simulink model "sim_bank_and_economy"  (R2020a)
settings: Solver=VariableStepAuto  StartTime=0.0  StopTime=10.0  RelTol=1e-3
values from neighbouring files (symbols this model uses):
  c_fi = 0.5    [a_1.m]    (also in a_2.m; a_loss_function.m; bank_and_economy.m = 0.25)
  i_k = 0.06    [a_1.m]    (also in a_loss_function.m = 0.04; bank_and_economy.m = 0.04; full_model.m = 0.04)
  i_l = 0.075    [bank_and_economy.m]    (also in bank_centralbank.m = 0.055; bootstrapping.m = 0.055; main.m = 0.055)
  i_m = 0.03    [bank_and_economy.m]    (also in bank_centralbank.m; bootstrapping.m; main.m)
  K_0 = 0.08    [a_1.m]    (also in a_2.m; a_loss_function.m; bank_and_economy.m; bank_centralbank.m)
  K_p = 15    [a_1.m]    (also in a_2.m; a_loss_function.m; bank_and_economy.m = 0.5; bank_centralbank.m)
  l_k = 0.005    [bank_and_economy.m]
  lambda = 0.002    [a_1.m]    (also in a_2.m; a_loss_function.m; bank_and_economy.m; bank_centralbank.m)
  R = 1    [a_1.m]    (also in a_2.m; a_loss_function.m; bank_and_economy.m; bank_centralbank.m)
  r_k = 0.1    [a_1.m]    (also in a_2.m; a_loss_function.m; bank_and_economy.m; full_model.m)
  rate = 0.1    [a_1.m]    (also in a_2.m; a_loss_function.m; bank_and_economy.m; bank_centralbank.m)
  s_kf = 0.75    [bank_and_economy.m]
  sigma = 0.28    [a_1.m]    (also in a_2.m; a_loss_function.m; bank_and_economy.m; bank_centralbank.m)
  start_f = temp    (= 1)    [bank_and_economy.m]    (also in economy.m = 100)
  start_g = temp    (= 1)    [bank_and_economy.m]    (also in economy.m = 100)
  start_h = temp    (= 1)    [bank_and_economy.m]    (also in economy.m = 100)
  T_f = 0.5    [a_1.m]    (also in a_2.m; a_loss_function.m; bank_and_economy.m; bank_centralbank.m)
  T_g = 1    [a_1.m]    (also in a_2.m; a_loss_function.m; bank_and_economy.m; bank_centralbank.m)
  T_h = 0.1    [a_1.m]    (also in a_2.m; a_loss_function.m; bank_and_economy.m; bank_centralbank.m)
  T_i = 8    [a_1.m]    (also in a_2.m; a_loss_function.m; bank_and_economy.m; bank_centralbank.m)
  T_k = 0.1    [a_1.m]    (also in a_2.m; a_loss_function.m; bank_and_economy.m = 0.25; economy.m = 1)
  T_kf = 0.25    [bank_and_economy.m]
  tx = 0.3    [a_1.m]    (also in a_2.m; a_loss_function.m; bank_and_economy.m = 0.5; bank_centralbank.m = 0.25)
settings Model: Creator=erlended  LastModifiedBy=erlended

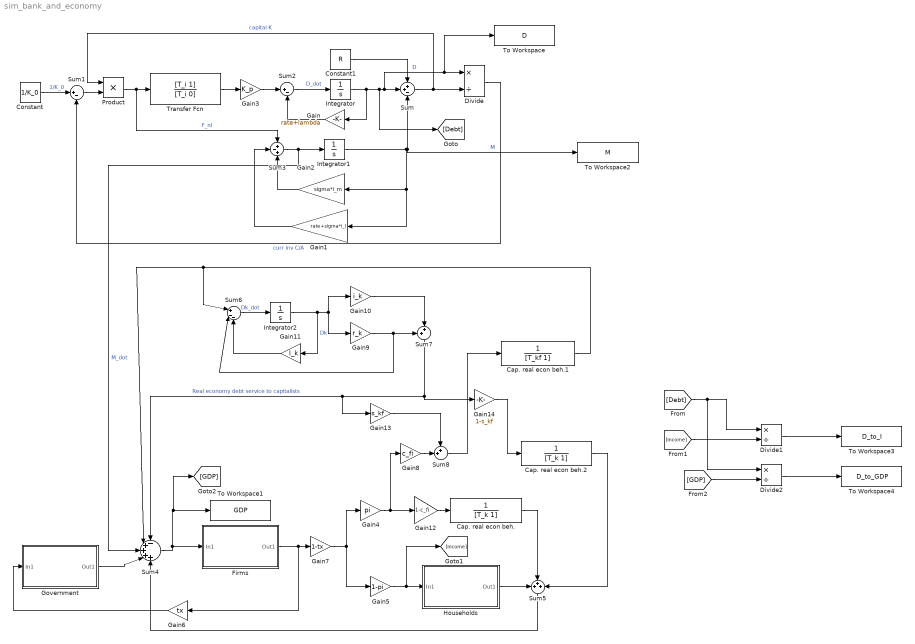
== system sim_bank_and_economy ==
  Cap. real econ beh. : TransferFcn  Denominator=[T_k 1]
  Cap. real econ beh.1 : TransferFcn  Denominator=[T_kf 1]
  Cap. real econ beh.2 : TransferFcn  Denominator=[T_k 1]
  Constant : Constant  Value=1/K_0
  Constant1 : Constant  Value=R
  Divide : Product  Inputs=*/
  Divide1 : Product  Inputs=*/
  Divide2 : Product  Inputs=*/
  Firms : Subsystem
  Gain : Gain  Gain=rate+lambda
  Gain1 : Gain  Gain=rate+sigma*i_l
  Gain10 : Gain  Gain=i_k
  Gain11 : Gain  Gain=l_k
  Gain12 : Gain  Gain=1-c_fi
  Gain13 : Gain  Gain=s_kf
  Gain14 : Gain  Gain=1-s_kf
  Gain2 : Gain  Gain=sigma*i_m
  Gain3 : Gain  Gain=K_p
  Gain4 : Gain  Gain=pi
  Gain5 : Gain  Gain=1-pi
  Gain6 : Gain  Gain=tx
  Gain7 : Gain  Gain=1-tx
  Gain8 : Gain  Gain=c_fi
  Gain9 : Gain  Gain=r_k
  Government : Subsystem
  Households : Subsystem
  Integrator : Integrator
  Integrator1 : Integrator
  Integrator2 : Integrator
  Product : Product
  Sum : Sum  Inputs=++-
  Sum1 : Sum  Inputs=|+-
  Sum2 : Sum  Inputs=|+-
  Sum3 : Sum  Inputs=+-+
  Sum4 : Sum  Inputs=-++++
  Sum5 : Sum  Inputs=+++
  Sum6 : Sum  Inputs=|+--
  Sum7 : Sum  Inputs=++|
  Sum8 : Sum  Inputs=++|
  To Workspace : ToWorkspace  VariableName=D  SaveFormat=Timeseries  SampleTime=-1
  To Workspace1 : ToWorkspace  VariableName=GDP  SaveFormat=Timeseries  SampleTime=-1
  To Workspace2 : ToWorkspace  VariableName=M  SaveFormat=Timeseries  SampleTime=-1
  To Workspace3 : ToWorkspace  VariableName=D_to_I  SaveFormat=Timeseries  SampleTime=-1
  To Workspace4 : ToWorkspace  VariableName=D_to_GDP  SaveFormat=Timeseries  SampleTime=-1
  Transfer Fcn : TransferFcn  Numerator=[T_i 1]  Denominator=[T_i 0]
  wires:
  Gain3/1 -> Sum2/1
  Integrator/1 -> Gain/1, [Debt], To Workspace/1, Divide/1, Sum/2  "D"
  Transfer Fcn/1 -> Gain3/1
  Divide/1 -> Sum1/2  "curr inv C/A"
  Gain1/1 -> Sum3/2
  Gain2/1 -> Sum3/3
  Sum1/1 -> Product/2
  Constant/1 -> Sum1/1  "1/K_0"
  Integrator1/1 -> Gain1/1, Gain2/1, To Workspace2/1, Sum/3  "M"
  Sum3/1 -> Sum4/3, Integrator1/1  "M_dot"
  Sum2/1 -> Integrator/1  "D_dot"
  Gain/1 -> Sum2/2
  Constant1/1 -> Sum/1
  Sum/1 -> Product/1, Divide/2  "capital K"
  Product/1 -> Transfer Fcn/1, Sum3/1  "F_nl"
  Households/1(Out1) -> Sum5/1
  Gain7/1 -> Gain4/1, Gain5/1
  Sum4/1 -> Firms/1(In1), [GDP], To Workspace1/1
  Sum5/1 -> Sum4/5
  Gain6/1 -> Government/1(In1)
  Firms/1(Out1) -> Gain7/1, Gain6/1
  Government/1(Out1) -> Sum4/4
  Gain5/1 -> [Income], Households/1(In1)
  Cap. real econ beh./1 -> Sum5/2
  Divide1/1 -> To Workspace3/1
  Divide2/1 -> To Workspace4/1
  [Debt] -> Divide1/1, Divide2/1
  [GDP] -> Divide2/2
  [Income] -> Divide1/2
  Integrator2/1 -> Gain11/1, Gain9/1, Gain10/1  "Dk"
  Sum6/1 -> Integrator2/1  "Dk_dot"
  Gain11/1 -> Sum6/3
  Gain10/1 -> Sum7/2
  Gain9/1 -> Sum6/2, Sum7/1
  Sum7/1 -> Gain14/1, Sum4/1, Gain13/1  "Real economy debt service to capitalists"
  Gain4/1 -> Gain12/1, Gain8/1
  Gain12/1 -> Cap. real econ beh./1
  Gain8/1 -> Sum8/2
  Sum8/1 -> Cap. real econ beh.1/1
  Cap. real econ beh.1/1 -> Sum4/2, Sum6/1
  Gain13/1 -> Sum8/1
  Gain14/1 -> Cap. real econ beh.2/1
  Cap. real econ beh.2/1 -> Sum5/3

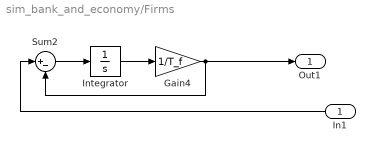
== system sim_bank_and_economy/Firms ==
  In1 : Inport
  Gain4 : Gain  Gain=1/T_f
  Integrator : Integrator  InitialCondition=start_f
  Sum2 : Sum  Inputs=|+-
  Out1 : Outport
  wires:
  In1/1 -> Sum2/1
  Sum2/1 -> Integrator/1
  Gain4/1 -> Out1/1, Sum2/2
  Integrator/1 -> Gain4/1

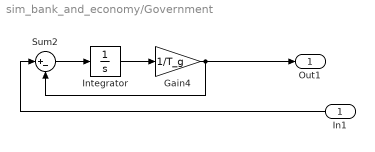
== system sim_bank_and_economy/Government ==
  In1 : Inport
  Gain4 : Gain  Gain=1/T_g
  Integrator : Integrator  InitialCondition=start_g
  Sum2 : Sum  Inputs=|+-
  Out1 : Outport
  wires:
  In1/1 -> Sum2/1
  Sum2/1 -> Integrator/1
  Gain4/1 -> Out1/1, Sum2/2
  Integrator/1 -> Gain4/1

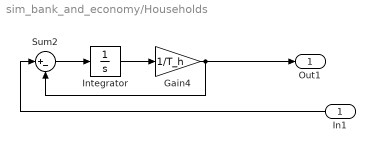
== system sim_bank_and_economy/Households ==
  In1 : Inport
  Gain4 : Gain  Gain=1/T_h
  Integrator : Integrator  InitialCondition=start_h
  Sum2 : Sum  Inputs=|+-
  Out1 : Outport
  wires:
  In1/1 -> Sum2/1
  Sum2/1 -> Integrator/1
  Gain4/1 -> Out1/1, Sum2/2
  Integrator/1 -> Gain4/1
